simulink model "Zustandsregelung_mit_Vorsteuerung_nichtlinear"  (R2021b)
settings: Solver=FixedStepAuto  StartTime=0.0  StopTime=25  FixedStep=1/1e4  RelTol=1e-3
undefined symbols (not defined in the file): F, k_Vorsteuerung, start_deg, x_Ruhe, y_ref
settings Model: Creator=basti  LastModifiedBy=aaron

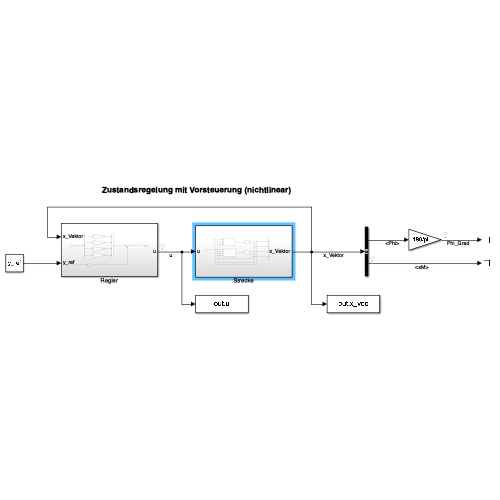
[thumbnail: Simulink's stored preview of the top-level diagram]
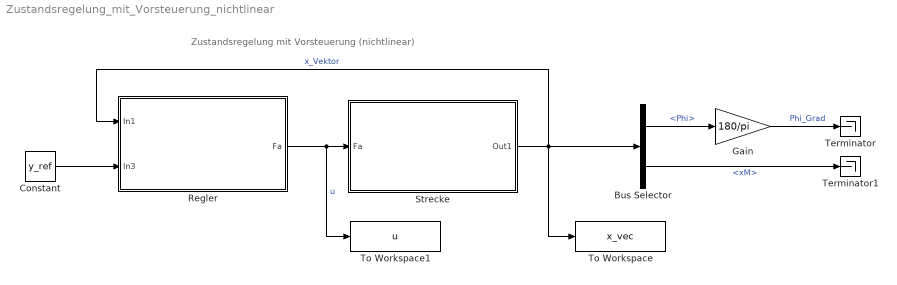
== system Zustandsregelung_mit_Vorsteuerung_nichtlinear ==
  note: Zustandsregelung mit Vorsteuerung (nichtlinear)
  Bus Selector : BusSelector  OutputSignals=Phi,xM
  Constant : Constant  Value=y_ref
  Gain : Gain  Gain=180/pi
  Regler : Subsystem
  Strecke : Subsystem
  Terminator : Terminator
  Terminator1 : Terminator
  To Workspace : ToWorkspace  VariableName=x_vec  SaveFormat=Timeseries  SampleTime=-1
  To Workspace1 : ToWorkspace  VariableName=u  SaveFormat=Timeseries  SampleTime=-1
  wires:
  Gain/1 -> Terminator/1  "Phi_Grad"
  Bus Selector/2 -> Terminator1/1  "<xM>"
  Strecke/1(Out1) -> To Workspace/1, Regler/1(In1), Bus Selector/1  "x_Vektor"
  Bus Selector/1 -> Gain/1  "<Phi>"
  Regler/1(Fa) -> To Workspace1/1, Strecke/1(Fa)  "u"
  Constant/1 -> Regler/2(In3)

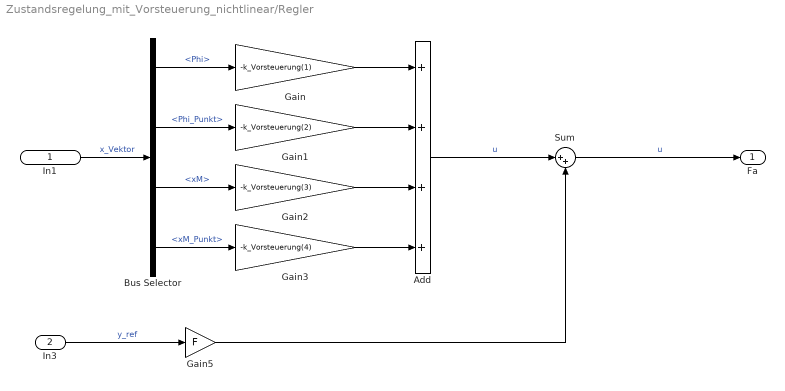
== system Zustandsregelung_mit_Vorsteuerung_nichtlinear/Regler ==
  In1 : Inport
  In3 : Inport  Port=2
  Add : Sum  Inputs=++++
  Bus Selector : BusSelector  OutputSignals=Phi,Phi_Punkt,xM,xM_Punkt
  Gain : Gain  Gain=-k_Vorsteuerung(1)
  Gain1 : Gain  Gain=-k_Vorsteuerung(2)
  Gain2 : Gain  Gain=-k_Vorsteuerung(3)
  Gain3 : Gain  Gain=-k_Vorsteuerung(4)
  Gain5 : Gain  Gain=F
  Sum : Sum  Inputs=|++
  Fa : Outport
  wires:
  Gain2/1 -> Add/3
  Gain1/1 -> Add/2
  Gain/1 -> Add/1
  Gain3/1 -> Add/4
  In1/1 -> Bus Selector/1  "x_Vektor"
  Bus Selector/1 -> Gain/1  "<Phi>"
  Bus Selector/2 -> Gain1/1  "<Phi_Punkt>"
  Bus Selector/3 -> Gain2/1  "<xM>"
  Bus Selector/4 -> Gain3/1  "<xM_Punkt>"
  Gain5/1 -> Sum/2
  In3/1 -> Gain5/1  "y_ref"
  Sum/1 -> Fa/1  "u"
  Add/1 -> Sum/1  "u"

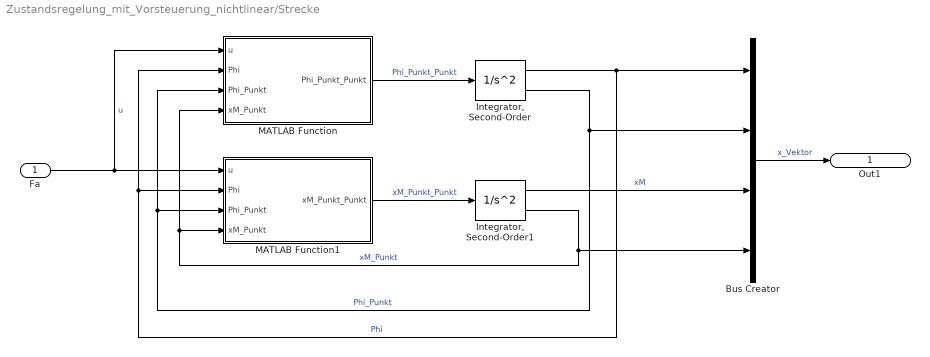
== system Zustandsregelung_mit_Vorsteuerung_nichtlinear/Strecke ==
  Fa : Inport
  Bus Creator : BusCreator  Inputs=4
  "Integrator, Second-Order" : SecondOrderIntegrator  ICX=(start_deg*pi)/180  ICDXDT=x_Ruhe(2, 1)
  "Integrator, Second-Order1" : SecondOrderIntegrator  ICX=x_Ruhe(3, 1)  ICDXDT=x_Ruhe(4, 1)
  MATLAB Function : MATLAB Function  TreatAsAtomicUnit=on
  MATLAB Function1 : MATLAB Function  TreatAsAtomicUnit=on
  Out1 : Outport
  wires:
  "Integrator, Second-Order1"/2 -> Bus Creator/4, MATLAB Function1/4(xM_Punkt), MATLAB Function/4(xM_Punkt)  "xM_Punkt"
  "Integrator, Second-Order"/1 -> Bus Creator/1, MATLAB Function/2(Phi), MATLAB Function1/2(Phi)  "Phi"
  "Integrator, Second-Order"/2 -> Bus Creator/2, MATLAB Function/3(Phi_Punkt), MATLAB Function1/3(Phi_Punkt)  "Phi_Punkt"
  Fa/1 -> MATLAB Function/1(u), MATLAB Function1/1(u)  "u"
  MATLAB Function/1(Phi_Punkt_Punkt) -> "Integrator, Second-Order"/1  "Phi_Punkt_Punkt"
  MATLAB Function1/1(xM_Punkt_Punkt) -> "Integrator, Second-Order1"/1  "xM_Punkt_Punkt"
  "Integrator, Second-Order1"/1 -> Bus Creator/3  "xM"
  Bus Creator/1 -> Out1/1  "x_Vektor"

== matlab function Zustandsregelung_mit_Vorsteuerung_nichtlinear/Strecke/MATLAB Function1 ==
  data: u input; xM_Punkt_Punkt output; Phi input; Phi_Punkt input; xM_Punkt input
function xM_Punkt_Punkt = fcn(u, Phi, Phi_Punkt, xM_Punkt)
    % Konstanten
    c = Konstanten();

    % Berechnung
    xM_Punkt_Punkt = (c.g*tan(Phi)+1/(c.m*cos(Phi)^2)*(c.d*xM_Punkt-u)-(c.l*Phi_Punkt^2*tan(Phi))/cos(Phi)-(c.d_Mf*Phi_Punkt)/(c.m*c.l*cos(Phi)))/(1-(c.M+c.m)/(c.m*cos(Phi)^2));

== matlab function Zustandsregelung_mit_Vorsteuerung_nichtlinear/Strecke/MATLAB Function ==
  data: u input; Phi_Punkt_Punkt output; Phi input; Phi_Punkt input; xM_Punkt input
function Phi_Punkt_Punkt = fcn(u, Phi, Phi_Punkt, xM_Punkt)
    % Konstanten
    c = Konstanten();

    % Berechnung
    Phi_Punkt_Punkt = ((u-c.g*tan(Phi)*(c.M+c.m)-c.d*xM_Punkt)/(c.m*c.l*cos(Phi))+c.d_Mf*Phi_Punkt*(c.M/(c.m^2*c.l^2*cos(Phi)^2)+1/(c.m*c.l^2*cos(Phi)^2))+Phi_Punkt^2*tan(Phi))/(1-(1/cos(Phi)^2)-c.M/(c.m*cos(Phi)^2));
